simulink model "EPS"  (R2020b)
settings: Solver=VariableStepAuto  StartTime=0.0  StopTime=60000  RelTol=1e-6
libraries: nesl_utility x4, fl_lib x4, ee_lib x1
settings Model: DataTypeOverride=Double  MinMaxOverflowLogging=ForceOff  PacingRate=100  Creator=abelaguiera  LastModifiedBy=abelaguilera

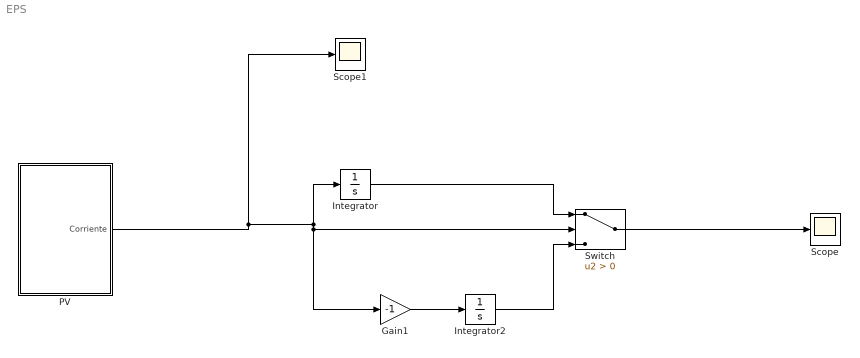
== system EPS ==
  Gain1 : Gain  Gain=-1
  Integrator : Integrator
  Integrator2 : Integrator
  PV : Subsystem
  Scope : Scope
  Scope1 : Scope
  Switch : Switch  Criteria=u2 > Threshold
  wires:
  Switch/1 -> Scope/1
  Integrator/1 -> Switch/1
  Integrator2/1 -> Switch/3
  PV/1(Corriente) -> Scope1/1, Gain1/1, Switch/2, Integrator/1
  Gain1/1 -> Integrator2/1

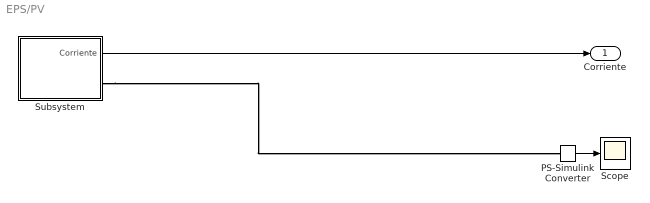
== system EPS/PV ==
  PS-Simulink Converter : nesl_utility/PS-Simulink Converter  PhysicalDomain=network_engine_domain  SubClassName=ps_output  LeftPortType=input  RightPortType=output  PseudoPeriodic=off  Frequencies=[]  Unit=inherit  AffineConversion=off
  Scope : Scope
  Subsystem : Subsystem
  Corriente : Outport
  wires:
  Subsystem/1(Corriente) -> Corriente/1
  PS-Simulink Converter/1 -> Scope/1
  connections:
  Subsystem/RConn1 -- PS-Simulink Converter/LConn1

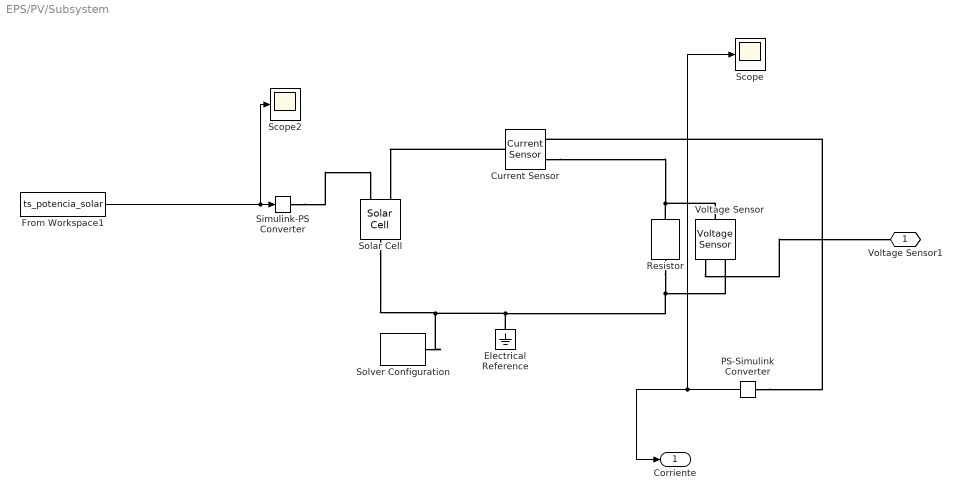
== system EPS/PV/Subsystem ==
  Current Sensor : fl_lib/Electrical/Electrical Sensors/Current Sensor
  Electrical Reference : fl_lib/Electrical/Electrical Elements/Electrical Reference
  From Workspace1 : FromWorkspace  VariableName=ts_potencia_solar
  PS-Simulink Converter : nesl_utility/PS-Simulink Converter  PhysicalDomain=network_engine_domain  SubClassName=ps_output  LeftPortType=input  RightPortType=output  PseudoPeriodic=off  Frequencies=[]  Unit=inherit  AffineConversion=off
  Resistor : fl_lib/Electrical/Electrical Elements/Resistor  R=10 Ohm  i_specify=off  i_priority=None  i=0 A  i_nominal_specify=off  i_nominal_unit=A  i_nominal_value=1  v_specify=off  v_priority=None  v=0 V  v_nominal_specify=off  v_nominal_unit=V  v_nominal_value=1
  Scope : Scope
  Scope2 : Scope
  Simulink-PS Converter : nesl_utility/Simulink-PS Converter  PhysicalDomain=network_engine_domain  SubClassName=ps_input  LeftPortType=input  RightPortType=output  PseudoPeriodic=off  Frequencies=[]  NoiseDistribution=none  NoiseParameters=[]  Unit=1  AffineConversion=off  FilteringAndDerivatives=provide  SimscapeFilterOrder=1  InputFilterTimeConstant=0.001  UdotUserProvided=0
  Solar Cell : ee_lib/Sources/Solar Cell  prm=1  Isc=4.35 A  Voc=0.6 V  Is=1e-6 A  Is2=0 A  Iph=8.217 A  Ir0=1000 W/m^2  ec=1.5  N2=2  Rs=0 Ohm  Rp=415 Ohm  N_series=36  TIPH1=0 1/K  EG=1.11 eV  TXIS1=3  TXIS2=3  TRS1=0  TRP1=0  Tmeas=25 degC  TFIXED=25 degC  thermal_mass=100 J/K  initial_temperature=25 degC
      settings: SourceProductBaseCode=PS
  Solver Configuration : nesl_utility/Solver Configuration  PhysicalDomain=network_engine_domain  SubClassName=solver  LeftPortType=input  RightPortType=generic  Tones=[]  Harmonics=[]  SimulateNoise=off  Profile=off  UseLocalSampling=off  EnableSwitchedLinearOptims=on  FrequencyDomain=off  UseCCode=off  RelTol=0.001  AbsTol=1e-06  MinStep=1e-09  ToWorkspace=off  RevertToSquareIcSolve=off  NumHomotopyIterations=100  PhasorMode=off  PhasorModeNumHarmonics=1  DoDC=on  ResidualTolerance=1e-09  UseLocalSolver=off  LocalSolverChoice=NE_BACKWARD_EULER_ADVANCER  LocalSolverSampleTime=0.001  DoFixedCost=off  MaxNonlinIter=3  MaxModeIter=2  ComputeImpulses=off  ImpulseIterations=2  LinearAlgebra=auto  EquationFormulation=NE_TIME_EF  DelaysMemoryBudget=1024  AutomaticFiltering=on  FilteringTimeConstant=0.001  PartitionStorageMethod=AS_NEEDED  PartitionMemoryBudget=1024  PartitionMethod=ROBUST
  Voltage Sensor : fl_lib/Electrical/Electrical Sensors/Voltage Sensor
  Voltage Sensor1 : PMIOPort  Side=Right
  Corriente : Outport
  wires:
  PS-Simulink Converter/1 -> Corriente/1, Scope/1
  From Workspace1/1 -> Scope2/1, Simulink-PS Converter/1
  connections:
  Simulink-PS Converter/RConn1 -- Solar Cell/LConn1
  Voltage Sensor/RConn1 -- Voltage Sensor1/RConn1
  Current Sensor/LConn1 -- Solar Cell/LConn2
  PS-Simulink Converter/LConn1 -- Current Sensor/RConn1
  Solar Cell/RConn1 -- Electrical Reference/LConn1 -- Resistor/RConn1 -- Voltage Sensor/RConn2 -- Solver Configuration/RConn1
  Current Sensor/RConn2 -- Resistor/LConn1 -- Voltage Sensor/LConn1
